simulink model "app_ComMgr"  (R2016b)
settings: Solver=FixedStepDiscrete  StartTime=0.0  StopTime=10.0  FixedStep=0.001  RelTol=1e-3  EnableMultiTasking=on
PreLoadFcn:
  | try
  |    tapas_types('load');
  | catch
  |   disp('TAPAS WARNING: Tapas Types could not be loaded ...');
  | end
  | 
  | try
  |   app_types('load');
  | catch
  |   currdir =pwd;
  |   try
  |     cd('..\app_types\');
  |     app_types('load');
  |     cd(currdir);
  |   catch
  |     try
  |        cd('..\..\app_types\');
  |        app_types('load');
  |        cd(currdir);
  |     catch
  |        cd(currdir);
  |        disp('TAPAS WARNING: Application Types could not be loaded ...');
  |     end
  |   end
  |   try
  |       clear currdir;
  |   catch
  |      %Do nothing
  |   end
  | end
libraries: Lib_v1p0_DE_ECU_Com x3
settings Model: Creator=kmansour  LastModifiedBy=kmansour
settings DataIOCC: LimitDataPoints=on  SaveFormat=Array
settings OptimizationCC: LifeSpan=1
settings DebuggingCC: AllowSymbolicDim=off  SFUnexpectedBacktrackingDiag=warning  SFNoUnconditionalDefaultTransitionDiag=warning  SFExecutionAtInitializationDiag=none
settings HardwareCC: ProdBitPerPointer=32  ProdBitPerSizeT=32  ProdBitPerPtrDiffT=32  ProdLargestAtomicInteger=Long  ProdLargestAtomicFloat=Double  ProdWordSize=32  ProdHWDeviceType=Texas Instruments->TMS570 Cortex-R4
settings ModelReferenceCC: ModelReferenceNumInstancesAllowed=Single  PropagateSignalLabelsOutOfModel=off
settings RTWCC: SystemTargetFile=ert.tlc  GenCodeOnly=on  TemplateMakefile=ert_default_tmf  Description=Embedded Coder  GenerateReport=on  IncludeHyperlinkInReport=on  LaunchReport=on  GenerateTraceInfo=on  GenerateTraceReport=on  GenerateTraceReportSl=on  GenerateTraceReportSf=on  GenerateTraceReportEml=on
settings CodeAppCC: IgnoreCustomStorageClasses=off  MaxIdLength=63
settings ERTTargetCC: GenerateSampleERTMain=on  ERTSrcFileBannerTemplate=tapas_code_template.cgt  ERTHdrFileBannerTemplate=tapas_code_template.cgt  ERTDataSrcFileTemplate=tapas_code_template.cgt  ERTDataHdrFileTemplate=tapas_code_template.cgt  ERTCustomFileTemplate=example_file_process.tlc  ConvertIfToSwitch=off  SuppressUnreachableDefaultCases=off
settings ConfigComp: CovMetricSettings=dw  CovHtmlReporting=on  CovSaveCumulativeToWorkspaceVar=on  CovSaveSingleToWorkspaceVar=on  CovExternalEMLEnable=off

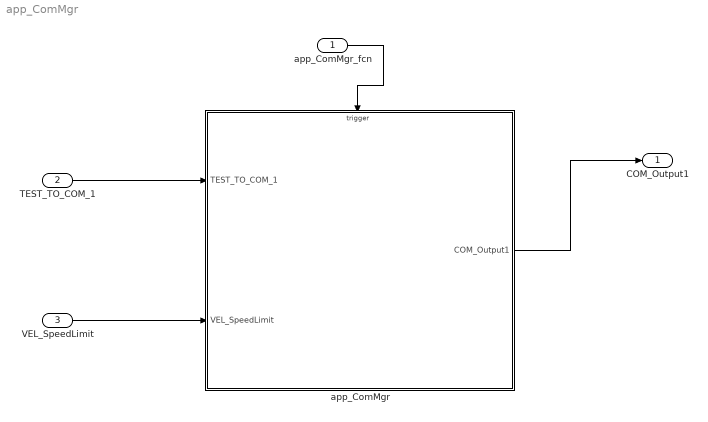
== system app_ComMgr ==
  app_ComMgr_fcn : Inport  SampleTime=100e-3  OutputFunctionCall=on
  TEST_TO_COM_1 : Inport  Port=2
  VEL_SpeedLimit : Inport  Port=3
  app_ComMgr : Subsystem
  COM_Output1 : Outport
  wires:
  app_ComMgr_fcn/1 -> app_ComMgr/Trigger
  TEST_TO_COM_1/1 -> app_ComMgr/1(TEST_TO_COM_1)
  app_ComMgr/1(COM_Output1) -> COM_Output1/1
  VEL_SpeedLimit/1 -> app_ComMgr/2(VEL_SpeedLimit)

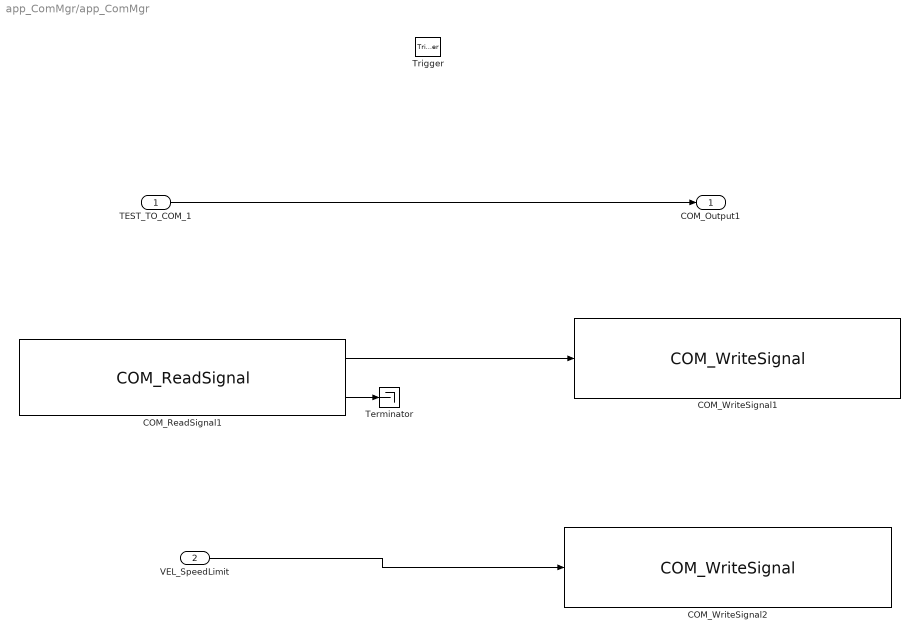
== system app_ComMgr/app_ComMgr ==
  TEST_TO_COM_1 : Inport
  VEL_SpeedLimit : Inport  Port=2
  Trigger : TriggerPort  TriggerType=function-call  VariantControl=Variant  SampleTimeType=periodic  SampleTime=-1  PortDimensions=1
  COM_ReadSignal1 : Lib_v1p0_DE_ECU_Com/COM_ReadSignal  PARAM_ID=APP_RX_VCU_VEHICLESPEED
  COM_WriteSignal1 : Lib_v1p0_DE_ECU_Com/COM_WriteSignal  PARAM_ID=APP_TX_ME_SPEED
  COM_WriteSignal2 : Lib_v1p0_DE_ECU_Com/COM_WriteSignal  PARAM_ID=APP_TX_DE_CONTROL_SPEEDSETPOINT
  Terminator : Terminator
  COM_Output1 : Outport
  wires:
  TEST_TO_COM_1/1 -> COM_Output1/1
  COM_ReadSignal1/2 -> Terminator/1
  COM_ReadSignal1/1 -> COM_WriteSignal1/1
  VEL_SpeedLimit/1 -> COM_WriteSignal2/1
